simulink model "shake_table"  (R2018b)
settings: Solver=VariableStepAuto  StartTime=0.0  StopTime=1  RelTol=1e-3
libraries: simulink x1
settings Model: Creator=EMiR  LastModifiedBy=EMiR

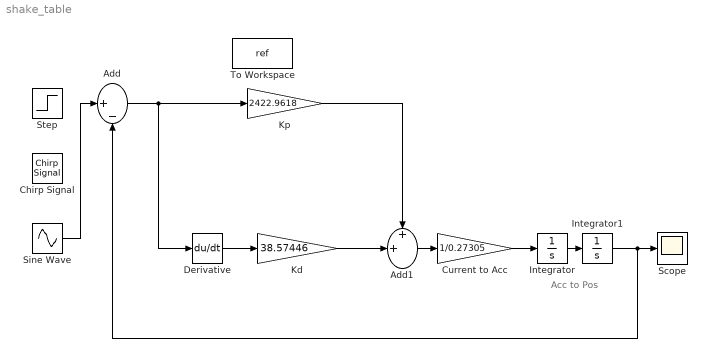
== system shake_table ==
  note: Acc to Pos
  Add : Sum  Inputs=|+-
  Add1 : Sum  Inputs=++|
  Chirp Signal : simulink/Sources/Chirp Signal  f1=0.1  T=20  f2=30
  "Current to Acc " : Gain  Gain=1/0.27305
  Derivative : Derivative
  Integrator : Integrator
  Integrator1 : Integrator
  Kd : Gain  Gain=38.57446
  "Kp " : Gain  Gain=2422.9618
  Scope : Scope
  Sine Wave : Sin  Frequency=32  SampleTime=0
  Step : Step  Time=0  SampleTime=0
  To Workspace : ToWorkspace  VariableName=ref  SampleTime=-1
  wires:
  Kd/1 -> Add1/2
  Add1/1 -> "Current to Acc "/1
  "Kp "/1 -> Add1/1
  Add/1 -> Derivative/1, "Kp "/1
  Integrator/1 -> Integrator1/1
  "Current to Acc "/1 -> Integrator/1
  Integrator1/1 -> Scope/1, Add/2
  Derivative/1 -> Kd/1
  Sine Wave/1 -> Add/1
